simulink model "TwoSegmentArm_muscles_v002"  (R2024b)
settings: Solver=VariableStepAuto  StartTime=0.0  StopTime=20  RelTol=1e-3  AbsTol=1e-3  EnableMultiTasking=on
model workspace (MAT data in the model file):
  bp_out = [-2.4 1.9]
values from neighbouring files (symbols this model uses):
  Param_Mus_MEE = Library_mtu_simulink_mtu_standard_parameters(Param_Mus_MEE)    [init_muscle_MEE.m]
  Param_Mus_MEF = Library_mtu_simulink_mtu_standard_parameters(Param_Mus_MEF)    [init_muscle_MEF.m]
  Param_Mus_MSA = Library_mtu_simulink_mtu_standard_parameters(Param_Mus_MSA)    [init_muscle_MSA.m]
  Param_Mus_MSR = Library_mtu_simulink_mtu_standard_parameters(Param_Mus_MSR)    [init_muscle_MSR.m]
  random_offset = 0    [ddpg_agent.m]
  Ts = 0.075    [ddpg_agent.m]
undefined symbols (not defined in the file or in its folder): gaussian, X, Y, Z
libraries: sm_lib x22, nesl_utility x15, Library_mtu_simulink x8, simulink x8, rllib x1
settings Model: Creator=Isabell  LastModifiedBy=morit
settings SolverCC: AutoScaleAbsTol=off  AlgebraicLoopSolver=TrustRegion
settings DataIOCC: LimitDataPoints=on  MaxDataPoints=10000
settings OptimizationCC: LifeSpan=inf
settings DebuggingCC: UnconnectedInputMsg=warning  UnconnectedOutputMsg=warning  UnconnectedLineMsg=warning  AllowSymbolicDim=off  SFUnexpectedBacktrackingDiag=warning  SFNoUnconditionalDefaultTransitionDiag=warning  SFExecutionAtInitializationDiag=none  ArithmeticOperatorsInVariantConditions=warning
settings ModelReferenceCC: EnableRefExpFcnMdlSchedulingChecks=on
settings SFSimCC: SimUseLocalCustomCode=off  CustomCodeUndefinedFunction=UseInterfaceOnly
settings RTWCC: RTWUseLocalCustomCode=off  GPUComputeCapability=3.5  DLArmComputeVersion=19.05
settings CodeAppCC: StateflowObjectComments=on
settings GRTTargetCC: TargetLangStandard=C89/C90 (ANSI)
settings ConfigComp: CovMetricSettings=dw  CovSaveCumulativeToWorkspaceVar=on  CovSaveSingleToWorkspaceVar=on  CovExternalEMLEnable=off  CovSFcnEnable=off
settings SimscapeCC: SimscapeLogType=all  SimscapeLogSimulationStatistics=on  SimscapeLogDataHistory=10000

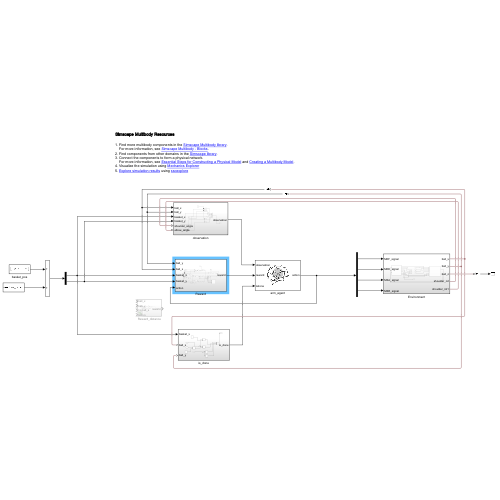
[thumbnail: Simulink's stored preview of the top-level diagram]
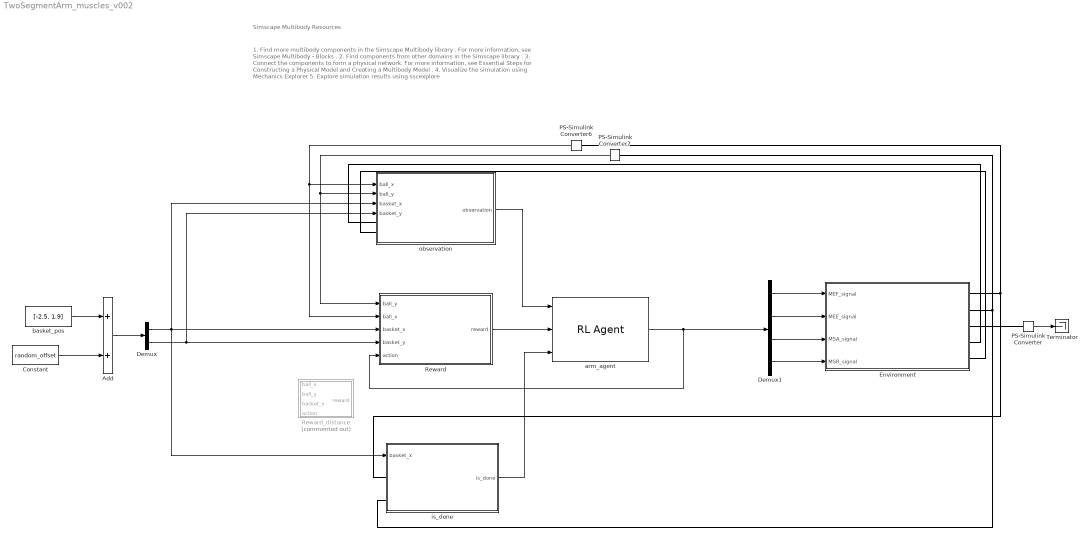
== system TwoSegmentArm_muscles_v002 ==
  note: 1. Find more multibody components in the Simscape Multibody library .
      | For more information, see Simscape Multibody - Blocks .
      | 2. Find components from other domains in the Simscape library .
      | 3. Connect the components to form a physical network.
      | For more information, see Essential Steps for Constructing a Physical Model and Creating a Multibody Model .
      | 4. Visualize the simulation using Mechanics Explorer
      | 5. Explore simulation results using sscexplore
  note: Simscape Multibody Resources
  Add : Sum
  Constant : Constant  Value=random_offset
  Demux : Demux  Outputs=2
  Demux1 : Demux
  Environment : Subsystem
  PS-Simulink Converter : nesl_utility/PS-Simulink Converter  PhysicalDomain=network_engine_domain  SubClassName=ps_output  LeftPortType=input  RightPortType=output  PseudoPeriodic=off  Frequencies=[]  VectorFormat=inherit  Unit=inherit  AffineConversion=off
  PS-Simulink Converter6 : nesl_utility/PS-Simulink Converter  PhysicalDomain=network_engine_domain  SubClassName=ps_output  LeftPortType=input  RightPortType=output  PseudoPeriodic=off  Frequencies=[]  VectorFormat=inherit  Unit=inherit  AffineConversion=off
  PS-Simulink Converter7 : nesl_utility/PS-Simulink Converter  PhysicalDomain=network_engine_domain  SubClassName=ps_output  LeftPortType=input  RightPortType=output  PseudoPeriodic=off  Frequencies=[]  VectorFormat=inherit  Unit=inherit  AffineConversion=off
  Reward : Subsystem
  Reward_distance : Subsystem  Commented=on
  Terminator : Terminator
  arm_agent : rllib/RL Agent  Agent=agent  ExternalActionAsInput=off  ProvideLastAction=off  ProvideCumRwd=off  TreatAsDirectFeedthrough=on  UseStrictObservationDataTypes=off
  basket_pos : Constant  Value=[-2.5, 1.9]
  is_done : Subsystem
  observation : Subsystem
  wires:
  basket_pos/1 -> Add/1
  Add/1 -> Demux/1
  Demux1/3 -> Environment/3(MSA_signal)
  Demux1/2 -> Environment/2(MEE_signal)
  Constant/1 -> Add/2
  Demux1/1 -> Environment/1(MEF_signal)
  Demux1/4 -> Environment/4(MSR_signal)
  PS-Simulink Converter/1 -> Terminator/1
  observation/1(observation) -> arm_agent/1
  Demux/2 -> observation/4(basket_y), Reward/4(basket_y)
  Demux/1 -> Reward/3(basket_x), observation/3(basket_x), is_done/1(basket_x)
  is_done/1(is_done) -> arm_agent/3
  Reward/1(reward) -> arm_agent/2
  PS-Simulink Converter7/1 -> observation/2(ball_y), Reward/1(ball_y)
  arm_agent/1 -> Reward/5(action), Demux1/1
  PS-Simulink Converter6/1 -> Reward/2(ball_x), observation/1(ball_x)
  connections:
  Environment/RConn3 -- PS-Simulink Converter/LConn1
  Environment/RConn5 -- observation/LConn2
  Environment/RConn4 -- observation/LConn1
  Environment/RConn1 -- PS-Simulink Converter6/LConn1 -- is_done/LConn1
  PS-Simulink Converter7/LConn1 -- is_done/LConn2 -- Environment/RConn2

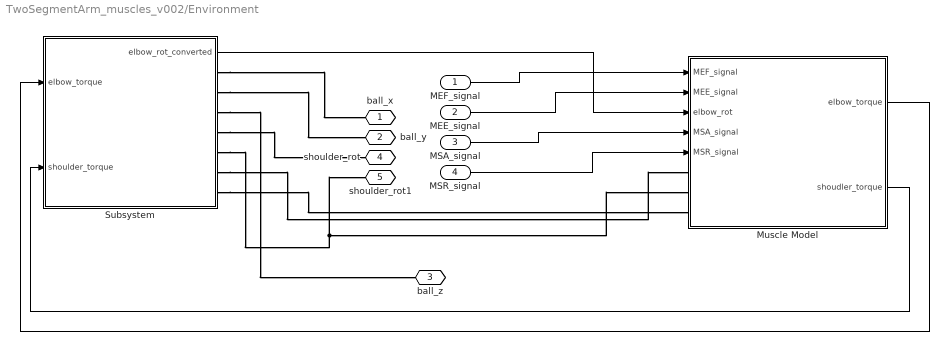
== system TwoSegmentArm_muscles_v002/Environment ==
  MEF_signal : Inport
  MEE_signal : Inport  Port=2
  MSA_signal : Inport  Port=3
  MSR_signal : Inport  Port=4
  Muscle Model : Subsystem
  Subsystem : Subsystem
  ball_x : PMIOPort  Side=Right
  ball_y : PMIOPort  Port=2  Side=Right
  ball_z : PMIOPort  Port=3  Side=Right
  shoulder_rot : PMIOPort  Port=4  Side=Right
  shoulder_rot1 : PMIOPort  Port=5  Side=Right
  wires:
  Muscle Model/2(shoudler_torque) -> Subsystem/2(shoulder_torque)
  Subsystem/1(elbow_rot_converted) -> Muscle Model/3(elbow_rot)
  MEF_signal/1 -> Muscle Model/1(MEF_signal)
  Muscle Model/1(elbow_torque) -> Subsystem/1(elbow_torque)
  MSA_signal/1 -> Muscle Model/4(MSA_signal)
  MSR_signal/1 -> Muscle Model/5(MSR_signal)
  MEE_signal/1 -> Muscle Model/2(MEE_signal)
  connections:
  Subsystem/RConn7 -- Muscle Model/LConn3
  Subsystem/RConn5 -- shoulder_rot1/RConn1 -- Muscle Model/LConn2
  Subsystem/RConn3 -- ball_z/RConn1
  Subsystem/RConn2 -- ball_y/RConn1
  Subsystem/RConn6 -- Muscle Model/LConn1
  Subsystem/RConn1 -- ball_x/RConn1
  Subsystem/RConn4 -- shoulder_rot/RConn1

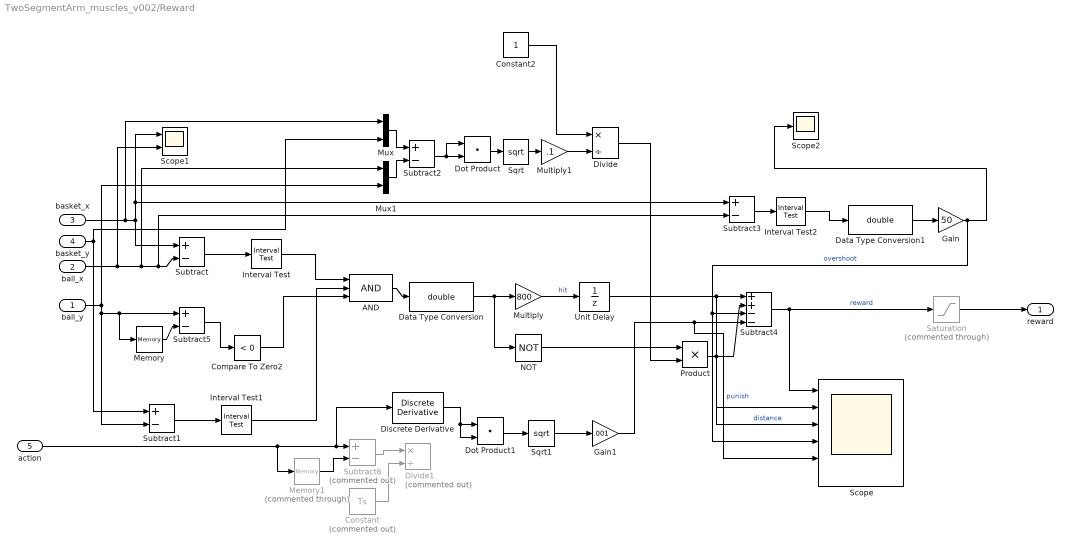
== system TwoSegmentArm_muscles_v002/Reward ==
  ball_y : Inport
  ball_x : Inport  Port=2
  basket_x : Inport  Port=3
  basket_y : Inport  Port=4
  action : Inport  Port=5
  AND : Logic  Inputs=3  IconShape=distinctive  AllPortsSameDT=off  OutDataTypeStr=boolean
  Compare To Zero2 : simulink/Logic and Bit Operations/Compare To Zero  relop=<  OutDataTypeStr=boolean
  Constant : Constant  Commented=on  Value=Ts
  Constant2 : Constant
  Data Type Conversion : DataTypeConversion  OutDataTypeStr=double  SaturateOnIntegerOverflow=off  RndMeth=Floor
  Data Type Conversion1 : DataTypeConversion  OutDataTypeStr=double  SaturateOnIntegerOverflow=off  RndMeth=Floor
  Discrete Derivative : simulink/Discrete/Discrete Derivative  gainval=1.0  ICPrevScaledInput=0.0  OutMin=[]  OutMax=[]  OutDataType=fixdt(1, 16)  OutScaling=2^-10  DoSatur=off
  Divide : Product  Inputs=*/
  Divide1 : Product  Commented=on  Inputs=*/
  Dot Product : DotProduct  OutDataTypeStr=Inherit: Inherit via internal rule
  Dot Product1 : DotProduct  OutDataTypeStr=Inherit: Inherit via internal rule
  Gain : Gain  Gain=50
  Gain1 : Gain  Gain=.001
  Interval Test : simulink/Logic and Bit Operations/Interval Test  IntervalClosedRight=on  uplimit=0.25  IntervalClosedLeft=on  lowlimit=-0.25  OutDataTypeStr=boolean
  Interval Test1 : simulink/Logic and Bit Operations/Interval Test  IntervalClosedRight=on  uplimit=0.05  IntervalClosedLeft=on  lowlimit=-0.25  OutDataTypeStr=boolean
  Interval Test2 : simulink/Logic and Bit Operations/Interval Test  IntervalClosedRight=on  uplimit=0.85  IntervalClosedLeft=on  lowlimit=0.25  OutDataTypeStr=boolean
  Memory : Memory
  Memory1 : Memory  Commented=through
  Multiply : Gain  Gain=800
  Multiply1 : Gain  Gain=.1
  Mux : Mux  Inputs=2
  Mux1 : Mux  Inputs=2
  NOT : Logic  Operator=NOT  IconShape=distinctive  AllPortsSameDT=off  OutDataTypeStr=boolean
  Product : Product
  Saturation : Saturate  Commented=through  UpperLimit=1500  LowerLimit=-500
  Scope : Scope  NumInputPorts=6
  Scope1 : Scope  NumInputPorts=2
  Scope2 : Scope
  Sqrt : Sqrt
  Sqrt1 : Sqrt
  Subtract{,1..3,5} (5 alike) : Sum  Inputs=+-
  Subtract4 : Sum  Inputs=++--
  Subtract6 : Sum  Commented=on  Inputs=+-
  Unit Delay : UnitDelay  SampleTime=-1  HasFrameUpgradeWarning=on
  reward : Outport
  wires:
  basket_x/1 -> Mux/1, Subtract/1, Subtract3/1, Scope1/1
  ball_x/1 -> Scope1/2, Mux1/1, Subtract3/2, Subtract/2
  Subtract/1 -> Interval Test/1
  ball_y/1 -> Subtract1/2, Memory/1, Subtract5/1, Mux1/2
  Subtract5/1 -> Compare To Zero2/1
  basket_y/1 -> Subtract1/1, Mux/2
  AND/1 -> Data Type Conversion/1
  NOT/1 -> Product/1
  Multiply/1 -> Unit Delay/1  "hit"
  Product/1 -> Subtract4/2, Scope/3  "distance"
  Subtract4/1 -> Saturation/1, Scope/1  "reward"
  Data Type Conversion/1 -> NOT/1, Multiply/1
  Interval Test/1 -> AND/1
  Subtract1/1 -> Interval Test1/1
  Interval Test1/1 -> AND/2
  Mux/1 -> Subtract2/1
  Mux1/1 -> Subtract2/2
  Subtract2/1 -> Dot Product/2, Dot Product/1
  Dot Product/1 -> Sqrt/1
  Sqrt/1 -> Multiply1/1
  Subtract3/1 -> Interval Test2/1
  Interval Test2/1 -> Data Type Conversion1/1
  Data Type Conversion1/1 -> Gain/1
  Gain/1 -> Scope/4, Subtract4/3, Scope2/1  "overshoot"
  Dot Product1/1 -> Sqrt1/1
  Gain1/1 -> Scope/5, Subtract4/4  "punish"
  Constant2/1 -> Divide/1
  Multiply1/1 -> Divide/2
  Divide/1 -> Product/2
  Sqrt1/1 -> Gain1/1
  Unit Delay/1 -> Scope/2, Subtract4/1
  Compare To Zero2/1 -> AND/3
  Memory/1 -> Subtract5/2
  Saturation/1 -> reward/1
  action/1 -> Memory1/1, Discrete Derivative/1, Subtract6/1
  Subtract6/1 -> Divide1/1
  Memory1/1 -> Subtract6/2
  Constant/1 -> Divide1/2
  Discrete Derivative/1 -> Dot Product1/2, Dot Product1/1

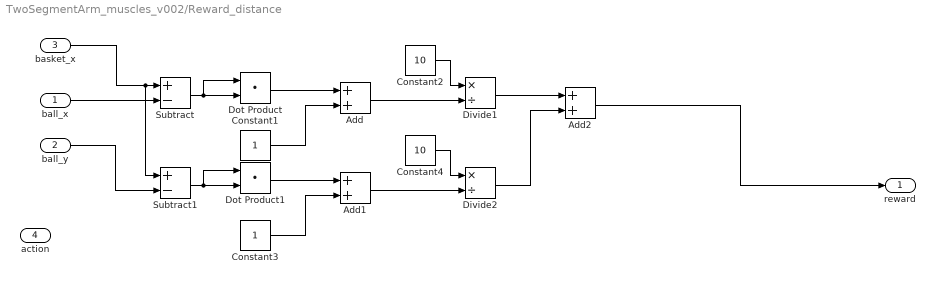
== system TwoSegmentArm_muscles_v002/Reward_distance ==
  ball_x : Inport
  ball_y : Inport  Port=2
  basket_x : Inport  Port=3
  action : Inport  Port=4
  Add : Sum
  Add1 : Sum
  Add2 : Sum
  Constant1 : Constant
  Constant2 : Constant  Value=10
  Constant3 : Constant
  Constant4 : Constant  Value=10
  Divide1 : Product  Inputs=*/
  Divide2 : Product  Inputs=*/
  Dot Product : DotProduct  OutDataTypeStr=Inherit: Inherit via internal rule
  Dot Product1 : DotProduct  OutDataTypeStr=Inherit: Inherit via internal rule
  Subtract : Sum  Inputs=+-
  Subtract1 : Sum  Inputs=+-
  reward : Outport
  wires:
  Add/1 -> Divide1/2
  Constant2/1 -> Divide1/1
  Subtract/1 -> Dot Product/1, Dot Product/2
  ball_x/1 -> Subtract/2
  Dot Product/1 -> Add/1
  Constant1/1 -> Add/2
  basket_x/1 -> Subtract1/1, Subtract/1
  Divide1/1 -> Add2/1
  Add1/1 -> Divide2/2
  Constant4/1 -> Divide2/1
  Dot Product1/1 -> Add1/1
  Subtract1/1 -> Dot Product1/1, Dot Product1/2
  Constant3/1 -> Add1/2
  Add2/1 -> reward/1
  Divide2/1 -> Add2/2
  ball_y/1 -> Subtract1/2

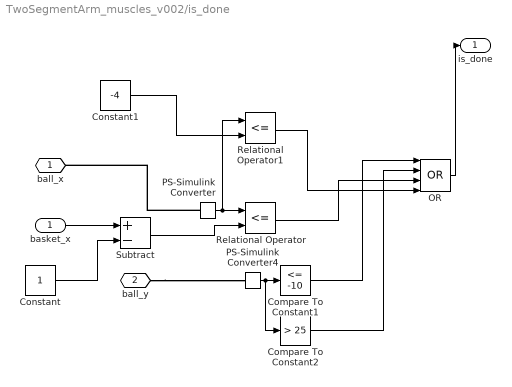
== system TwoSegmentArm_muscles_v002/is_done ==
  basket_x : Inport
  Compare To Constant1 : simulink/Logic and Bit Operations/Compare To Constant  relop=<=  const=-10  OutDataTypeStr=boolean
  Compare To Constant2 : simulink/Logic and Bit Operations/Compare To Constant  relop=>  const=25  OutDataTypeStr=boolean
  Constant : Constant
  Constant1 : Constant  Value=-4
  OR : Logic  Operator=OR  Inputs=4  IconShape=distinctive  AllPortsSameDT=off  OutDataTypeStr=boolean
  PS-Simulink Converter : nesl_utility/PS-Simulink Converter  PhysicalDomain=network_engine_domain  SubClassName=ps_output  LeftPortType=input  RightPortType=output  PseudoPeriodic=off  Frequencies=[]  VectorFormat=inherit  Unit=inherit  AffineConversion=off
  PS-Simulink Converter4 : nesl_utility/PS-Simulink Converter  PhysicalDomain=network_engine_domain  SubClassName=ps_output  LeftPortType=input  RightPortType=output  PseudoPeriodic=off  Frequencies=[]  VectorFormat=inherit  Unit=inherit  AffineConversion=off
  Relational Operator : RelationalOperator  Operator=<=  OutDataTypeStr=boolean  RndMeth=Simplest  InputSameDT=off
  Relational Operator1 : RelationalOperator  Operator=<=  OutDataTypeStr=boolean  RndMeth=Simplest  InputSameDT=off
  Subtract : Sum  Inputs=+-
  ball_x : PMIOPort  Side=Left
  ball_y : PMIOPort  Port=2  Side=Left
  is_done : Outport
  wires:
  PS-Simulink Converter4/1 -> Compare To Constant2/1, Compare To Constant1/1
  Compare To Constant1/1 -> OR/1
  Compare To Constant2/1 -> OR/2
  OR/1 -> is_done/1
  PS-Simulink Converter/1 -> Relational Operator1/1, Relational Operator/1
  Relational Operator/1 -> OR/3
  Constant/1 -> Subtract/2
  Subtract/1 -> Relational Operator/2
  basket_x/1 -> Subtract/1
  Constant1/1 -> Relational Operator1/2
  Relational Operator1/1 -> OR/4
  connections:
  ball_y/RConn1 -- PS-Simulink Converter4/LConn1
  PS-Simulink Converter/LConn1 -- ball_x/RConn1

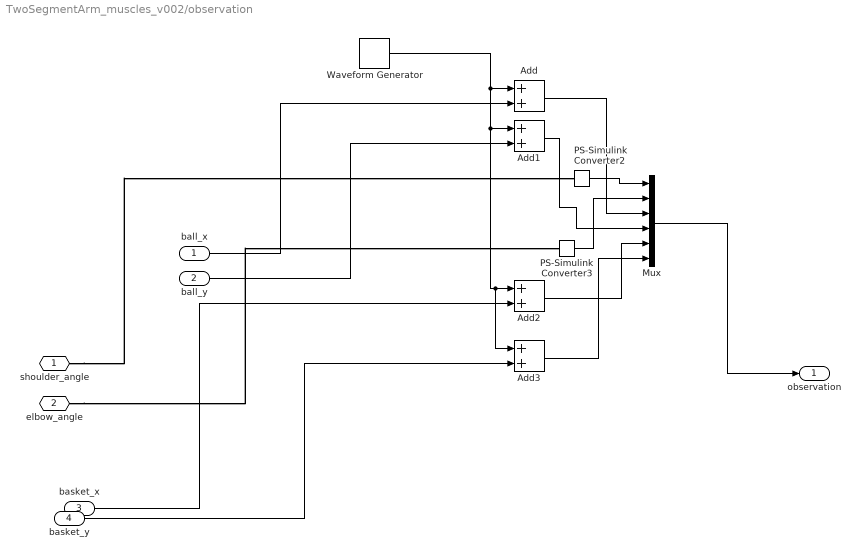
== system TwoSegmentArm_muscles_v002/observation ==
  ball_x : Inport
  ball_y : Inport  Port=2
  basket_x : Inport  Port=3
  basket_y : Inport  Port=4
  Add{,1..3} (4 alike) : Sum
  Mux : Mux  Inputs=6
  PS-Simulink Converter2 : nesl_utility/PS-Simulink Converter  PhysicalDomain=network_engine_domain  SubClassName=ps_output  LeftPortType=input  RightPortType=output  PseudoPeriodic=off  Frequencies=[]  VectorFormat=inherit  Unit=inherit  AffineConversion=off
  PS-Simulink Converter3 : nesl_utility/PS-Simulink Converter  PhysicalDomain=network_engine_domain  SubClassName=ps_output  LeftPortType=input  RightPortType=output  PseudoPeriodic=off  Frequencies=[]  VectorFormat=inherit  Unit=inherit  AffineConversion=off
  Waveform Generator : simulink/Sources/Waveform Generator  OutMin=[]  OutMax=[]  OutDataTypeStr=double  SelectedSignal=1  Signals=gaussian(0, 0, 120)  BlockNames=MultiportSwitch_2798d07791aa46f  SampleTime=0.1
  shoulder_angle : PMIOPort  Side=Left
  elbow_angle : PMIOPort  Port=2  Side=Left
  observation : Outport
  wires:
  Add/1 -> Mux/3
  Add1/1 -> Mux/4
  Waveform Generator/1 -> Add3/1, Add2/1, Add1/1, Add/1
  PS-Simulink Converter3/1 -> Mux/2
  Add3/1 -> Mux/6
  PS-Simulink Converter2/1 -> Mux/1
  Add2/1 -> Mux/5
  basket_y/1 -> Add3/2
  ball_x/1 -> Add/2
  Mux/1 -> observation/1
  ball_y/1 -> Add1/2
  basket_x/1 -> Add2/2
  connections:
  elbow_angle/RConn1 -- PS-Simulink Converter3/LConn1
  shoulder_angle/RConn1 -- PS-Simulink Converter2/LConn1

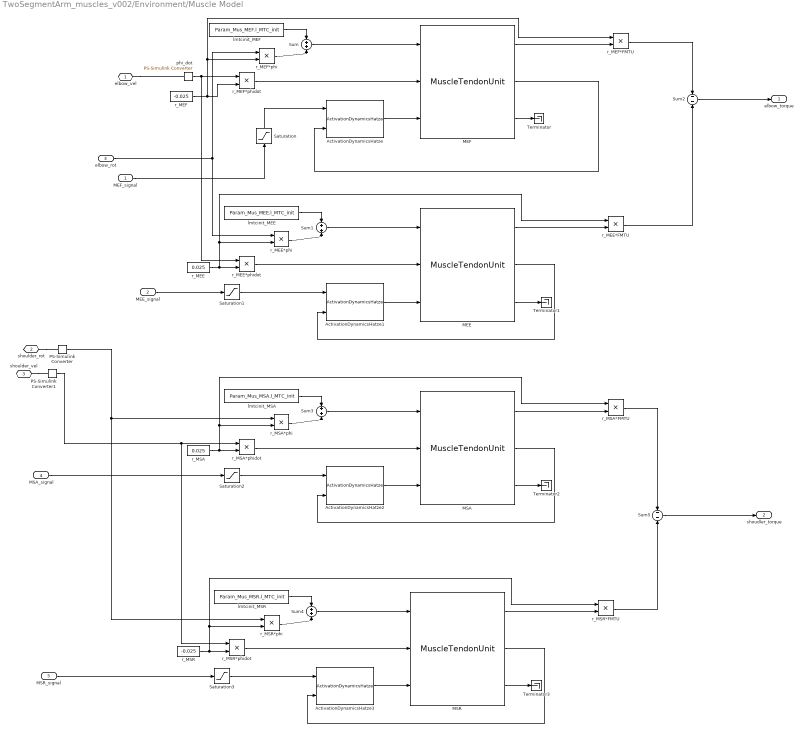
== system TwoSegmentArm_muscles_v002/Environment/Muscle Model ==
  MEF_signal : Inport
  MEE_signal : Inport  Port=2
  elbow_rot : Inport  Port=3
  MSA_signal : Inport  Port=4
  MSR_signal : Inport  Port=5
  ActivationDynamicsHatze : Library_mtu_simulink/ActivationDynamicsHatze  Act_Param=Param_Mus_MEF.ActDyn  Mus_Param=Param_Mus_MEF
  ActivationDynamicsHatze1 : Library_mtu_simulink/ActivationDynamicsHatze  Act_Param=Param_Mus_MEE.ActDyn  Mus_Param=Param_Mus_MEE
  ActivationDynamicsHatze2 : Library_mtu_simulink/ActivationDynamicsHatze  Act_Param=Param_Mus_MEE.ActDyn  Mus_Param=Param_Mus_MEE
  ActivationDynamicsHatze3 : Library_mtu_simulink/ActivationDynamicsHatze  Act_Param=Param_Mus_MEE.ActDyn  Mus_Param=Param_Mus_MEE
  MEE : Library_mtu_simulink/MuscleTendonUnit  Mus_Param=Param_Mus_MEE
  MEF : Library_mtu_simulink/MuscleTendonUnit  Mus_Param=Param_Mus_MEF
  MSA : Library_mtu_simulink/MuscleTendonUnit  Mus_Param=Param_Mus_MSA
  MSR : Library_mtu_simulink/MuscleTendonUnit  Mus_Param=Param_Mus_MSR
  PS-Simulink Converter : nesl_utility/PS-Simulink Converter  PhysicalDomain=network_engine_domain  SubClassName=ps_output  LeftPortType=input  RightPortType=output  PseudoPeriodic=off  Frequencies=[]  VectorFormat=inherit  Unit=inherit  AffineConversion=off
  PS-Simulink Converter1 : nesl_utility/PS-Simulink Converter  PhysicalDomain=network_engine_domain  SubClassName=ps_output  LeftPortType=input  RightPortType=output  PseudoPeriodic=off  Frequencies=[]  VectorFormat=inherit  Unit=inherit  AffineConversion=off
  Saturation{,1..3} (4 alike) : Saturate  UpperLimit=1  LowerLimit=0
  Sum{,1,3..4} (4 alike) : Sum  Inputs=+|+
  Sum2 : Sum  Inputs=-|-
  Sum5 : Sum  Inputs=-|-
  Terminator{,1..3} (4 alike) : Terminator
  lmtcinit_MEE : Constant  Value=Param_Mus_MEE.l_MTC_init
  lmtcinit_MEF : Constant  Value=Param_Mus_MEF.l_MTC_init
  lmtcinit_MSA : Constant  Value=Param_Mus_MSA.l_MTC_init
  lmtcinit_MSR : Constant  Value=Param_Mus_MSR.l_MTC_init
  phi_dot : nesl_utility/PS-Simulink Converter  PhysicalDomain=network_engine_domain  SubClassName=ps_output  LeftPortType=input  RightPortType=output  PseudoPeriodic=off  Frequencies=[]  VectorFormat=1-D array  Unit=inherit  AffineConversion=off
  r_MEE : Constant  Value=0.025
  r_MEE*FMTU : Product
  r_MEE*phi : Product
  r_MEE*phidot : Product
  r_MEF : Constant  Value=-0.025
  r_MEF*FMTU : Product
  r_MEF*phi : Product
  r_MEF*phidot : Product
  r_MSA : Constant  Value=0.025
  r_MSA*FMTU : Product
  r_MSA*phi : Product
  r_MSA*phidot : Product
  r_MSR : Constant  Value=-0.025
  r_MSR*FMTU : Product
  r_MSR*phi : Product
  r_MSR*phidot : Product
  elbow_vel : PMIOPort  Side=Left
  shoulder_rot : PMIOPort  Port=2  Side=Left
  shoulder_vel : PMIOPort  Port=3  Side=Left
  elbow_torque : Outport
  shoudler_torque : Outport  Port=2
  wires:
  Sum1/1 -> MEE/1
  MEE/3 -> Terminator1/1
  r_MEE*phi/1 -> Sum1/2
  elbow_rot/1 -> r_MEF*phi/1, r_MEE*phi/1
  r_MEF*phi/1 -> Sum/2
  r_MEF*phidot/1 -> MEF/2
  r_MEE/1 -> r_MEE*FMTU/1, r_MEE*phi/2, r_MEE*phidot/2
  MEF/3 -> Terminator/1
  r_MEE*FMTU/1 -> Sum2/2
  Saturation/1 -> ActivationDynamicsHatze/1
  MEE/1 -> r_MEE*FMTU/2
  r_MEF/1 -> r_MEF*FMTU/1, r_MEF*phi/2, r_MEF*phidot/2
  ActivationDynamicsHatze/1 -> MEF/3
  ActivationDynamicsHatze1/1 -> MEE/3
  Saturation1/1 -> ActivationDynamicsHatze1/1
  MEF/2 -> ActivationDynamicsHatze/2
  Sum/1 -> MEF/1
  MEF/1 -> r_MEF*FMTU/2
  MEE_signal/1 -> Saturation1/1
  phi_dot/1 -> r_MEE*phidot/1, r_MEF*phidot/1
  lmtcinit_MEF/1 -> Sum/1
  r_MEF*FMTU/1 -> Sum2/1
  r_MEE*phidot/1 -> MEE/2
  lmtcinit_MEE/1 -> Sum1/1
  MEE/2 -> ActivationDynamicsHatze1/2
  Sum2/1 -> elbow_torque/1
  MEF_signal/1 -> Saturation/1
  MSR/2 -> ActivationDynamicsHatze3/2
  MSR/1 -> r_MSR*FMTU/2
  r_MSR*FMTU/1 -> Sum5/2
  PS-Simulink Converter/1 -> r_MSR*phi/1, r_MSA*phi/1
  r_MSR*phi/1 -> Sum4/2
  PS-Simulink Converter1/1 -> r_MSR*phidot/1, r_MSA*phidot/1
  MSR/3 -> Terminator3/1
  ActivationDynamicsHatze3/1 -> MSR/3
  ActivationDynamicsHatze2/1 -> MSA/3
  Saturation3/1 -> ActivationDynamicsHatze3/1
  r_MSA*phidot/1 -> MSA/2
  r_MSR/1 -> r_MSR*FMTU/1, r_MSR*phi/2, r_MSR*phidot/2
  r_MSA*phi/1 -> Sum3/2
  Sum4/1 -> MSR/1
  MSA/2 -> ActivationDynamicsHatze2/2
  Sum3/1 -> MSA/1
  r_MSA*FMTU/1 -> Sum5/1
  Saturation2/1 -> ActivationDynamicsHatze2/1
  r_MSR*phidot/1 -> MSR/2
  MSA/3 -> Terminator2/1
  lmtcinit_MSR/1 -> Sum4/1
  lmtcinit_MSA/1 -> Sum3/1
  r_MSA/1 -> r_MSA*FMTU/1, r_MSA*phi/2, r_MSA*phidot/2
  MSA/1 -> r_MSA*FMTU/2
  MSA_signal/1 -> Saturation2/1
  MSR_signal/1 -> Saturation3/1
  Sum5/1 -> shoudler_torque/1
  connections:
  elbow_vel/RConn1 -- phi_dot/LConn1
  shoulder_rot/RConn1 -- PS-Simulink Converter/LConn1
  shoulder_vel/RConn1 -- PS-Simulink Converter1/LConn1

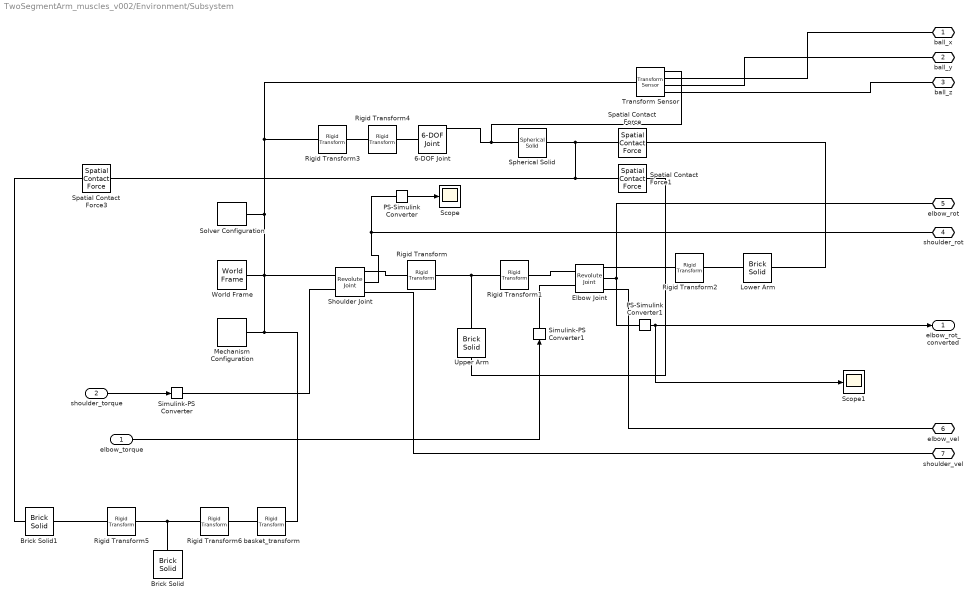
== system TwoSegmentArm_muscles_v002/Environment/Subsystem ==
  elbow_torque : Inport
  shoulder_torque : Inport  Port=2
  6-DOF Joint : sm_lib/Joints/6-DOF Joint  JointMode=Normal  CompositeWrenchDir=FollowerOnBase  CompositeWrenchFrame=BaseFrame  SenseConstraintForce=off  SenseConstraintTorque=off  SenseTotalForce=off  SenseTotalTorque=off  PxPositionTargetSpecify=off  PxPositionTargetPriority=High  PxPositionTargetValue=0  PxPositionTargetValueUnits=m  PxVelocityTargetSpecify=off  PxVelocityTargetPriority=High  PxVelocityTargetValue=0  PxVelocityTargetValueUnits=m/s  PxEquilibriumPosition=0  PxEquilibriumPositionUnits=m  PxSpringStiffness=0  PxSpringStiffnessUnits=N/m  PxDampingCoefficient=0  PxDampingCoefficientUnits=N/(m/s)  PxLowerLimitSpecify=off  PxLowerLimitBound=-1  PxLowerLimitBoundUnits=m  PxLowerLimitStiffness=1e6  PxLowerLimitStiffnessUnits=N/m  PxLowerLimitDamping=1e3  PxLowerLimitDampingUnits=N/(m/s)  PxLowerLimitTransitionRegionWidth=1e-4  PxLowerLimitTransitionRegionWidthUnits=m  PxUpperLimitSpecify=off  PxUpperLimitBound=1  PxUpperLimitBoundUnits=m  PxUpperLimitStiffness=1e6  PxUpperLimitStiffnessUnits=N/m  PxUpperLimitDamping=1e3  PxUpperLimitDampingUnits=N/(m/s)  PxUpperLimitTransitionRegionWidth=1e-4  PxUpperLimitTransitionRegionWidthUnits=m  PxTorqueActuationMode=NoTorque  PxMotionActuationMode=ComputedMotion  PxSensePosition=on  PxSenseVelocity=off  PxSenseAcceleration=off  PxSenseTorqueForce=off  PxSenseLowerLimitTorqueForce=off  PxSenseUpperLimitTorqueForce=off  PyPositionTargetSpecify=off  PyPositionTargetPriority=High  PyPositionTargetValue=0  PyPositionTargetValueUnits=m  PyVelocityTargetSpecify=off  PyVelocityTargetPriority=High  PyVelocityTargetValue=0  PyVelocityTargetValueUnits=m/s  PyEquilibriumPosition=0  PyEquilibriumPositionUnits=m  PySpringStiffness=0  PySpringStiffnessUnits=N/m  PyDampingCoefficient=0  PyDampingCoefficientUnits=N/(m/s)  PyLowerLimitSpecify=off  PyLowerLimitBound=-1  PyLowerLimitBoundUnits=m  PyLowerLimitStiffness=1e6  PyLowerLimitStiffnessUnits=N/m  PyLowerLimitDamping=1e3  PyLowerLimitDampingUnits=N/(m/s)  PyLowerLimitTransitionRegionWidth=1e-4  PyLowerLimitTransitionRegionWidthUnits=m  PyUpperLimitSpecify=off  PyUpperLimitBound=1  PyUpperLimitBoundUnits=m  PyUpperLimitStiffness=1e6  PyUpperLimitStiffnessUnits=N/m  PyUpperLimitDamping=1e3  PyUpperLimitDampingUnits=N/(m/s)  PyUpperLimitTransitionRegionWidth=1e-4  PyUpperLimitTransitionRegionWidthUnits=m  PyTorqueActuationMode=NoTorque  PyMotionActuationMode=ComputedMotion  PySensePosition=on  PySenseVelocity=off  PySenseAcceleration=off  PySenseTorqueForce=off  PySenseLowerLimitTorqueForce=off  PySenseUpperLimitTorqueForce=off  PzPositionTargetSpecify=off  PzPositionTargetPriority=High  PzPositionTargetValue=0  PzPositionTargetValueUnits=m  PzVelocityTargetSpecify=off  PzVelocityTargetPriority=High  PzVelocityTargetValue=0  PzVelocityTargetValueUnits=m/s  PzEquilibriumPosition=0  PzEquilibriumPositionUnits=m  PzSpringStiffness=0  PzSpringStiffnessUnits=N/m  PzDampingCoefficient=0  PzDampingCoefficientUnits=N/(m/s)  PzLowerLimitSpecify=off  PzLowerLimitBound=-1  PzLowerLimitBoundUnits=m  PzLowerLimitStiffness=1e6  PzLowerLimitStiffnessUnits=N/m  PzLowerLimitDamping=1e3  PzLowerLimitDampingUnits=N/(m/s)  PzLowerLimitTransitionRegionWidth=1e-4  PzLowerLimitTransitionRegionWidthUnits=m  PzUpperLimitSpecify=off  PzUpperLimitBound=1  PzUpperLimitBoundUnits=m  PzUpperLimitStiffness=1e6  PzUpperLimitStiffnessUnits=N/m  PzUpperLimitDamping=1e3  PzUpperLimitDampingUnits=N/(m/s)  PzUpperLimitTransitionRegionWidth=1e-4  PzUpperLimitTransitionRegionWidthUnits=m  PzTorqueActuationMode=NoTorque  PzMotionActuationMode=ComputedMotion  PzSensePosition=on  PzSenseVelocity=off  PzSenseAcceleration=off  PzSenseTorqueForce=off  PzSenseLowerLimitTorqueForce=off  PzSenseUpperLimitTorqueForce=off  SphPositionTargetSpecify=off  SphPositionTargetPriority=High  SphPositionTargetRotationMethod=None  SphPositionTargetFollAlignAxisA=+X  SphPositionTargetBaseAlignAxisA=+Y  SphPositionTargetFollAlignAxisB=+Y  SphPositionTargetBaseAlignAxisB=+Z  SphPositionTargetRotationStandardAxis=+Z  SphPositionTargetRotationAngle=0  SphPositionTargetRotationAngleUnits=deg  SphPositionTargetRotationArbitraryAxis=[0 0 1]  SphPositionTargetRotationSequenceAxes=FollowerAxes  SphPositionTargetRotationSequence=XYX  SphPositionTargetRotationSequenceAngles=[0 0 0]  SphPositionTargetRotationSequenceAnglesUnits=deg  SphPositionTargetRotationMatrix=[1 0 0;0 1 0;0 0 1]  SphPositionTargetQuaternion=[1 0 0 0]  SphVelocityTargetSpecify=off  SphVelocityTargetPriority=High  SphVelocityTargetValue=[0 0 0]  SphVelocityTargetValueUnits=deg/s  SphVelocityTargetInFollowerFrame=on  SphEqPosRotationMethod=None  SphEqPosFollAlignAxisA=+X  SphEqPosBaseAlignAxisA=+Y  SphEqPosFollAlignAxisB=+Y  SphEqPosBaseAlignAxisB=+Z  SphEqPosRotationStandardAxis=+Z  SphEqPosRotationAngle=0  SphEqPosRotationAngleUnits=deg  SphEqPosRotationArbitraryAxis=[0 0 1]  SphEqPosRotationSequenceAxes=FollowerAxes  SphEqPosRotationSequence=XYX  SphEqPosRotationSequenceAngles=[0 0 0]  SphEqPosRotationSequenceAnglesUnits=deg  SphEqPosRotationMatrix=[1 0 0;0 1 0;0 0 1]  SphEqPosQuaternion=[1 0 0 0]  SphSpringStiffness=0  SphSpringStiffnessUnits=N*m/deg  SphDampingCoefficient=0  SphDampingCoefficientUnits=N*m/(deg/s)  SphLowerLimitSpecify=off  SphLowerLimitBound=15  SphLowerLimitBoundUnits=deg  SphLowerLimitStiffness=1e4  SphLowerLimitStiffnessUnits=N*m/deg  SphLowerLimitDamping=10  SphLowerLimitDampingUnits=N*m/(deg/s)  SphLowerLimitTransitionRegionWidth=0.1  SphLowerLimitTransitionRegionWidthUnits=deg  SphUpperLimitSpecify=off  SphUpperLimitBound=45  SphUpperLimitBoundUnits=deg  SphUpperLimitStiffness=1e4  SphUpperLimitStiffnessUnits=N*m/deg  SphUpperLimitDamping=10  SphUpperLimitDampingUnits=N*m/(deg/s)  SphUpperLimitTransitionRegionWidth=0.1  SphUpperLimitTransitionRegionWidthUnits=deg  SphTorqueActuationMode=NoTorque  SphActuateTorqueX=off  SphActuateTorqueY=off  SphActuateTorqueZ=off  SphActuateTorque=off  SphActuationFrame=BaseFrame  SphSensePosition=off  SphSenseVelocityX=off  SphSenseVelocityY=off  SphSenseVelocityZ=off  SphSenseVelocity=off  SphSenseAccelerationX=off  SphSenseAccelerationY=off  SphSenseAccelerationZ=off  SphSenseAcceleration=off  SphSenseLowerLimitTorqueMag=off  SphSenseUpperLimitTorqueMag=off  SphSensingFrame=BaseFrame
  Brick Solid : sm_lib/Body Elements/Brick Solid  BrickDimensions=[.25 .05 .25]  BrickDimensionsUnits=m  ExportEntireGeometry=off  InertiaType=CalculateFromGeometry  BasedOnType=Density  Density=1000  DensityUnits=kg/m^3  Mass=1  MassUnits=kg  CenterOfMass=[0 0 0]  CenterOfMassUnits=m  MomentsOfInertia=[1 1 1]  MomentsOfInertiaUnits=kg*m^2  ProductsOfInertia=[0 0 0]  ProductsOfInertiaUnits=kg*m^2  GraphicType=FromGeometry  MarkerShape=Sphere  MarkerSize=10  GraphicVisPropType=SimpleVisualProperties  GraphicDiffuseColor=[0.5 0.5 0.5]  GraphicOpacity=1  GraphicSpecularColor=[0.5 0.5 0.5 1.0]  GraphicAmbientColor=[0.15 0.15 0.15 1.0]  GraphicEmissiveColor=[0.0 0.0 0.0 1.0]  GraphicShininess=75  DoExposeReferenceFrame=on  SerializedFrames=<Frames/>
  Brick Solid1 : sm_lib/Body Elements/Brick Solid  BrickDimensions=[.05 .3 .3]  BrickDimensionsUnits=m  ExportEntireGeometry=on  InertiaType=CalculateFromGeometry  BasedOnType=Density  Density=1000  DensityUnits=kg/m^3  Mass=1  MassUnits=kg  CenterOfMass=[0 0 0]  CenterOfMassUnits=m  MomentsOfInertia=[1 1 1]  MomentsOfInertiaUnits=kg*m^2  ProductsOfInertia=[0 0 0]  ProductsOfInertiaUnits=kg*m^2  GraphicType=FromGeometry  MarkerShape=Sphere  MarkerSize=10  GraphicVisPropType=SimpleVisualProperties  GraphicDiffuseColor=[0.5 0.5 0.5]  GraphicOpacity=1  GraphicSpecularColor=[0.5 0.5 0.5 1.0]  GraphicAmbientColor=[0.15 0.15 0.15 1.0]  GraphicEmissiveColor=[0.0 0.0 0.0 1.0]  GraphicShininess=75  DoExposeReferenceFrame=on  SerializedFrames=<Frames/>
  Elbow Joint : sm_lib/Joints/Revolute Joint  JointMode=Normal  CompositeWrenchDir=FollowerOnBase  CompositeWrenchFrame=BaseFrame  SenseConstraintForce=off  SenseConstraintTorque=off  SenseTotalForce=off  SenseTotalTorque=off  PositionTargetSpecify=on  PositionTargetPriority=High  PositionTargetValue=-130  PositionTargetValueUnits=deg  VelocityTargetSpecify=off  VelocityTargetPriority=High  VelocityTargetValue=0  VelocityTargetValueUnits=deg/s  EquilibriumPosition=0  EquilibriumPositionUnits=deg  SpringStiffness=0  SpringStiffnessUnits=N*m/deg  DampingCoefficient=0  DampingCoefficientUnits=N*m/(deg/s)  LowerLimitSpecify=on  LowerLimitBound=-135  LowerLimitBoundUnits=deg  LowerLimitStiffness=1000  LowerLimitStiffnessUnits=N*m/deg  LowerLimitDamping=10  LowerLimitDampingUnits=N*m/(rad/s)  LowerLimitTransitionRegionWidth=0.1  LowerLimitTransitionRegionWidthUnits=deg  UpperLimitSpecify=on  UpperLimitBound=0  UpperLimitBoundUnits=deg  UpperLimitStiffness=1000  UpperLimitStiffnessUnits=N*m/rad  UpperLimitDamping=10  UpperLimitDampingUnits=N*m/(rad/s)  UpperLimitTransitionRegionWidth=0.1  UpperLimitTransitionRegionWidthUnits=deg  TorqueActuationMode=InputTorque  MotionActuationMode=ComputedMotion  SensePosition=on  SenseVelocity=on  SenseAcceleration=off  SenseTorqueForce=off  SenseLowerLimitTorqueForce=off  SenseUpperLimitTorqueForce=off
  Lower Arm : sm_lib/Body Elements/Brick Solid  BrickDimensions=[0.01 0.263 0.01]  BrickDimensionsUnits=m  ExportEntireGeometry=on  InertiaType=Custom  BasedOnType=Density  Density=1000  DensityUnits=kg/m^3  Mass=1.65  MassUnits=kg  CenterOfMass=[0 -0.0475 0]  CenterOfMassUnits=m  MomentsOfInertia=[0 0 0.025]  MomentsOfInertiaUnits=kg*m^2  ProductsOfInertia=[0 0 0]  ProductsOfInertiaUnits=kg*m^2  GraphicType=FromGeometry  MarkerShape=Sphere  MarkerSize=10  GraphicVisPropType=SimpleVisualProperties  GraphicDiffuseColor=[0.0 0.0 1.0]  GraphicOpacity=1.0  GraphicSpecularColor=[0.5 0.5 0.5 1.0]  GraphicAmbientColor=[0.15 0.15 0.15 1.0]  GraphicEmissiveColor=[0.0 0.0 0.0 1.0]  GraphicShininess=75  DoExposeReferenceFrame=on  SerializedFrames=<Frames/>
  Mechanism Configuration : sm_lib/Utilities/Mechanism Configuration  UniformGravity=Constant  GravityVector=[0 -9.80665 0]  GravityVectorUnits=m/s^2  LinearizationDelta=0.001  JointModeTransitionNonlinearIterations=2
  PS-Simulink Converter : nesl_utility/PS-Simulink Converter  PhysicalDomain=network_engine_domain  SubClassName=ps_output  LeftPortType=input  RightPortType=output  PseudoPeriodic=off  Frequencies=[]  VectorFormat=1-D array  Unit=inherit  AffineConversion=off
  PS-Simulink Converter1 : nesl_utility/PS-Simulink Converter  PhysicalDomain=network_engine_domain  SubClassName=ps_output  LeftPortType=input  RightPortType=output  PseudoPeriodic=off  Frequencies=[]  VectorFormat=1-D array  Unit=inherit  AffineConversion=off
  Rigid Transform : sm_lib/Frames and Transforms/Rigid Transform  RotationMethod=None  FollAlignAxisA=+X  BaseAlignAxisA=+Y  FollAlignAxisB=+Y  BaseAlignAxisB=+Z  RotationStandardAxis=+Z  RotationAngle=0.0  RotationAngleUnits=deg  RotationArbitraryAxis=[0 0 1]  RotationSequenceAxes=FollowerAxes  RotationSequence=XYX  RotationSequenceAngles=[0 0 0]  RotationSequenceAnglesUnits=deg  RotationMatrix=[1 0 0; 0 1 0; 0 0 1]  Quaternion=[1 0 0 0]  TranslationMethod=StandardAxis  TranslationCartesianOffset=[0 0 0]  TranslationCartesianOffsetUnits=m  TranslationStandardAxis=+Y  TranslationStandardOffset=-0.1675  TranslationStandardOffsetUnits=m  TranslationROffset=0  TranslationROffsetUnits=m  TranslationThetaOffset=0  TranslationThetaOffsetUnits=deg  TranslationZOffset=0  TranslationZOffsetUnits=m
  Rigid Transform1 : sm_lib/Frames and Transforms/Rigid Transform  RotationMethod=None  FollAlignAxisA=+X  BaseAlignAxisA=+Y  FollAlignAxisB=+Y  BaseAlignAxisB=+Z  RotationStandardAxis=+Z  RotationAngle=0.0  RotationAngleUnits=deg  RotationArbitraryAxis=[0 0 1]  RotationSequenceAxes=FollowerAxes  RotationSequence=XYX  RotationSequenceAngles=[0 0 0]  RotationSequenceAnglesUnits=deg  RotationMatrix=[1 0 0; 0 1 0; 0 0 1]  Quaternion=[1 0 0 0]  TranslationMethod=StandardAxis  TranslationCartesianOffset=[0 0 0]  TranslationCartesianOffsetUnits=m  TranslationStandardAxis=+Y  TranslationStandardOffset=-0.1675  TranslationStandardOffsetUnits=m  TranslationROffset=0  TranslationROffsetUnits=m  TranslationThetaOffset=0  TranslationThetaOffsetUnits=deg  TranslationZOffset=0  TranslationZOffsetUnits=m
  Rigid Transform2 : sm_lib/Frames and Transforms/Rigid Transform  RotationMethod=None  FollAlignAxisA=+X  BaseAlignAxisA=+Y  FollAlignAxisB=+Y  BaseAlignAxisB=+Z  RotationStandardAxis=+Z  RotationAngle=0.0  RotationAngleUnits=deg  RotationArbitraryAxis=[0 0 1]  RotationSequenceAxes=FollowerAxes  RotationSequence=XYX  RotationSequenceAngles=[0 0 0]  RotationSequenceAnglesUnits=deg  RotationMatrix=[1 0 0; 0 1 0; 0 0 1]  Quaternion=[1 0 0 0]  TranslationMethod=StandardAxis  TranslationCartesianOffset=[0 0 0]  TranslationCartesianOffsetUnits=m  TranslationStandardAxis=+Y  TranslationStandardOffset=-0.1315  TranslationStandardOffsetUnits=m  TranslationROffset=0  TranslationROffsetUnits=m  TranslationThetaOffset=0  TranslationThetaOffsetUnits=deg  TranslationZOffset=0  TranslationZOffsetUnits=m
  Rigid Transform3 : sm_lib/Frames and Transforms/Rigid Transform  RotationMethod=None  FollAlignAxisA=+X  BaseAlignAxisA=+Y  FollAlignAxisB=+Y  BaseAlignAxisB=+Z  RotationStandardAxis=+Z  RotationAngle=0  RotationAngleUnits=deg  RotationArbitraryAxis=[0 0 1]  RotationSequenceAxes=FollowerAxes  RotationSequence=XYX  RotationSequenceAngles=[0 0 0]  RotationSequenceAnglesUnits=deg  RotationMatrix=[1 0 0;0 1 0;0 0 1]  Quaternion=[1 0 0 0]  TranslationMethod=StandardAxis  TranslationCartesianOffset=[0 0 0]  TranslationCartesianOffsetUnits=m  TranslationStandardAxis=+X  TranslationStandardOffset=0  TranslationStandardOffsetUnits=m  TranslationROffset=0  TranslationROffsetUnits=m  TranslationThetaOffset=0  TranslationThetaOffsetUnits=deg  TranslationZOffset=0  TranslationZOffsetUnits=m
  Rigid Transform4 : sm_lib/Frames and Transforms/Rigid Transform  RotationMethod=None  FollAlignAxisA=+X  BaseAlignAxisA=+Y  FollAlignAxisB=+Y  BaseAlignAxisB=+Z  RotationStandardAxis=+Z  RotationAngle=0  RotationAngleUnits=deg  RotationArbitraryAxis=[0 0 1]  RotationSequenceAxes=FollowerAxes  RotationSequence=XYX  RotationSequenceAngles=[0 0 0]  RotationSequenceAnglesUnits=deg  RotationMatrix=[1 0 0;0 1 0;0 0 1]  Quaternion=[1 0 0 0]  TranslationMethod=StandardAxis  TranslationCartesianOffset=[0 0 0]  TranslationCartesianOffsetUnits=m  TranslationStandardAxis=+Y  TranslationStandardOffset=.33  TranslationStandardOffsetUnits=m  TranslationROffset=0  TranslationROffsetUnits=m  TranslationThetaOffset=0  TranslationThetaOffsetUnits=deg  TranslationZOffset=0  TranslationZOffsetUnits=m
  Rigid Transform5 : sm_lib/Frames and Transforms/Rigid Transform  RotationMethod=None  FollAlignAxisA=+X  BaseAlignAxisA=+Y  FollAlignAxisB=+Y  BaseAlignAxisB=+Z  RotationStandardAxis=+Z  RotationAngle=0  RotationAngleUnits=deg  RotationArbitraryAxis=[0 0 1]  RotationSequenceAxes=FollowerAxes  RotationSequence=XYX  RotationSequenceAngles=[0 0 0]  RotationSequenceAnglesUnits=deg  RotationMatrix=[1 0 0;0 1 0;0 0 1]  Quaternion=[1 0 0 0]  TranslationMethod=Cartesian  TranslationCartesianOffset=[0.19, -0.15,0]  TranslationCartesianOffsetUnits=m  TranslationStandardAxis=-X  TranslationStandardOffset=.3  TranslationStandardOffsetUnits=m  TranslationROffset=0  TranslationROffsetUnits=m  TranslationThetaOffset=0  TranslationThetaOffsetUnits=deg  TranslationZOffset=0  TranslationZOffsetUnits=m
  Rigid Transform6 : sm_lib/Frames and Transforms/Rigid Transform  RotationMethod=None  FollAlignAxisA=+X  BaseAlignAxisA=+Y  FollAlignAxisB=+Y  BaseAlignAxisB=+Z  RotationStandardAxis=+Z  RotationAngle=0  RotationAngleUnits=deg  RotationArbitraryAxis=[0 0 1]  RotationSequenceAxes=FollowerAxes  RotationSequence=XYX  RotationSequenceAngles=[0 0 0]  RotationSequenceAnglesUnits=deg  RotationMatrix=[1 0 0;0 1 0;0 0 1]  Quaternion=[1 0 0 0]  TranslationMethod=StandardAxis  TranslationCartesianOffset=[0 0 0]  TranslationCartesianOffsetUnits=m  TranslationStandardAxis=-X  TranslationStandardOffset=random_offset  TranslationStandardOffsetUnits=m  TranslationROffset=0  TranslationROffsetUnits=m  TranslationThetaOffset=0  TranslationThetaOffsetUnits=deg  TranslationZOffset=0  TranslationZOffsetUnits=m
  Scope : Scope
  Scope1 : Scope
  Shoulder Joint : sm_lib/Joints/Revolute Joint  JointMode=Normal  CompositeWrenchDir=FollowerOnBase  CompositeWrenchFrame=BaseFrame  SenseConstraintForce=off  SenseConstraintTorque=off  SenseTotalForce=off  SenseTotalTorque=off  PositionTargetSpecify=on  PositionTargetPriority=High  PositionTargetValue=-140  PositionTargetValueUnits=deg  VelocityTargetSpecify=off  VelocityTargetPriority=High  VelocityTargetValue=0  VelocityTargetValueUnits=deg/s  EquilibriumPosition=0  EquilibriumPositionUnits=deg  SpringStiffness=0  SpringStiffnessUnits=N*m/deg  DampingCoefficient=0  DampingCoefficientUnits=N*m/(deg/s)  LowerLimitSpecify=on  LowerLimitBound=-180  LowerLimitBoundUnits=deg  LowerLimitStiffness=1000  LowerLimitStiffnessUnits=N*m/rad  LowerLimitDamping=10  LowerLimitDampingUnits=N*m/(rad/s)  LowerLimitTransitionRegionWidth=0.1  LowerLimitTransitionRegionWidthUnits=deg  UpperLimitSpecify=on  UpperLimitBound=0  UpperLimitBoundUnits=deg  UpperLimitStiffness=1000  UpperLimitStiffnessUnits=N*m/rad  UpperLimitDamping=10  UpperLimitDampingUnits=N*m/(rad/s)  UpperLimitTransitionRegionWidth=0.1  UpperLimitTransitionRegionWidthUnits=deg  TorqueActuationMode=InputTorque  MotionActuationMode=ComputedMotion  SensePosition=on  SenseVelocity=on  SenseAcceleration=off  SenseTorqueForce=off  SenseLowerLimitTorqueForce=off  SenseUpperLimitTorqueForce=off
  Simulink-PS Converter : nesl_utility/Simulink-PS Converter  PhysicalDomain=network_engine_domain  SubClassName=ps_input  LeftPortType=input  RightPortType=output  PseudoPeriodic=off  Frequencies=[]  NoiseDistribution=none  NoiseParameters=[]  Unit=1  AffineConversion=off  FilteringAndDerivatives=provide  SimscapeFilterOrder=1  InputFilterTimeConstant=0.001  UdotUserProvided=0
  Simulink-PS Converter1 : nesl_utility/Simulink-PS Converter  PhysicalDomain=network_engine_domain  SubClassName=ps_input  LeftPortType=input  RightPortType=output  PseudoPeriodic=off  Frequencies=[]  NoiseDistribution=none  NoiseParameters=[]  Unit=N*m  AffineConversion=off  FilteringAndDerivatives=provide  SimscapeFilterOrder=1  InputFilterTimeConstant=0.001  UdotUserProvided=0
  Solver Configuration : nesl_utility/Solver Configuration  PhysicalDomain=network_engine_domain  SubClassName=solver  LeftPortType=input  RightPortType=generic  Tones=[]  Harmonics=[]  SimulateNoise=off  Profile=off  UseLocalSampling=off  EnableSwitchedLinearOptims=on  FrequencyDomain=off  UseCCode=off  RelTol=0.001  AbsTol=1e-06  MinStep=1e-09  ToWorkspace=off  RevertToSquareIcSolve=off  NumHomotopyIterations=100  PhasorMode=off  PhasorModeNumHarmonics=1  ConsistencySolver=NEWTON_FTOL  IndexReductionMethod=DerivativeReplacement  DoDC=off  ResidualTolerance=1e-09  ConsistencyTolSource=GLOBAL  ConsistencyAbsTol=0.001  ConsistencyRelTol=0.001  ConsistencyTolFactor=0.001  UseLocalSolver=off  LocalSolverChoice=NE_BACKWARD_EULER_ADVANCER  ResolveIndetEquations=on  FunctionEvalNumThread=1  LocalSolverSampleTime=0.001  DoFixedCost=off  MaxNonlinIter=3  MaxModeIter=2  ComputeImpulses=off  ImpulseIterations=2  LinearAlgebra=Sparse  LinearAlgebraNumThread=0  EquationFormulation=NE_TIME_EF  DelaysMemoryBudget=1024  AutomaticFiltering=on  FilteringTimeConstant=0.001  PartitionStorageMethod=AS_NEEDED  PartitionMemoryBudget=1024  PartitionMethod=FAST  MultibodyUseLocalSolver=off  MultibodyLocalSolverChoice=ODE1  MultibodyLocalSolverSampleTime=0.001
  Spatial Contact Force : sm_lib/Forces and Torques/Spatial Contact Force  NormalForceType=SmoothSpringDamper  NormalStiffness=1e6  NormalStiffnessUnits=N/m  NormalDamping=1e3  NormalDampingUnits=N/(m/s)  NormalTransitionRegionWidth=1e-4  NormalTransitionRegionWidthUnits=m  FrictionType=SmoothStickSlip  CoefficientOfStaticFriction=0.5  CoefficientOfDynamicFriction=0.3  FrictionalCriticalVelocity=1e-3  FrictionalCriticalVelocityUnits=m/s  SenseContactSignal=off  SensePenetrationDepth=off  SenseSeparationDistance=off  SenseNormalForceMagnitude=off  SenseFrictionalForceMagnitude=off  SenseNormalVelocity=off  SenseTangentialVelocity=off  SenseContactBaseRotation=off  SenseContactBaseTranslation=off  SenseContactFollowerRotation=off  SenseContactFollowerTranslation=off  ZeroCrossDetectContactStartAndEnd=off
  Spatial Contact Force1 : sm_lib/Forces and Torques/Spatial Contact Force  NormalForceType=SmoothSpringDamper  NormalStiffness=1e6  NormalStiffnessUnits=N/m  NormalDamping=1e3  NormalDampingUnits=N/(m/s)  NormalTransitionRegionWidth=1e-4  NormalTransitionRegionWidthUnits=m  FrictionType=SmoothStickSlip  CoefficientOfStaticFriction=0.5  CoefficientOfDynamicFriction=0.3  FrictionalCriticalVelocity=1e-3  FrictionalCriticalVelocityUnits=m/s  SenseContactSignal=off  SensePenetrationDepth=off  SenseSeparationDistance=off  SenseNormalForceMagnitude=off  SenseFrictionalForceMagnitude=off  SenseNormalVelocity=off  SenseTangentialVelocity=off  SenseContactBaseRotation=off  SenseContactBaseTranslation=off  SenseContactFollowerRotation=off  SenseContactFollowerTranslation=off  ZeroCrossDetectContactStartAndEnd=off
  Spatial Contact Force3 : sm_lib/Forces and Torques/Spatial Contact Force  NormalForceType=SmoothSpringDamper  NormalStiffness=1e6  NormalStiffnessUnits=N/m  NormalDamping=1e3  NormalDampingUnits=N/(m/s)  NormalTransitionRegionWidth=1e-4  NormalTransitionRegionWidthUnits=m  FrictionType=SmoothStickSlip  CoefficientOfStaticFriction=0.5  CoefficientOfDynamicFriction=0.3  FrictionalCriticalVelocity=1e-3  FrictionalCriticalVelocityUnits=m/s  SenseContactSignal=off  SensePenetrationDepth=off  SenseSeparationDistance=off  SenseNormalForceMagnitude=off  SenseFrictionalForceMagnitude=off  SenseNormalVelocity=off  SenseTangentialVelocity=off  SenseContactBaseRotation=off  SenseContactBaseTranslation=off  SenseContactFollowerRotation=off  SenseContactFollowerTranslation=off  ZeroCrossDetectContactStartAndEnd=off
  Spherical Solid : sm_lib/Body Elements/Spherical Solid  SphereRadius=0.05  SphereRadiusUnits=m  ExportEntireGeometry=on  InertiaType=Custom  BasedOnType=Density  Density=1000  DensityUnits=kg/m^3  Mass=0.05  MassUnits=kg  CenterOfMass=[0 0 0]  CenterOfMassUnits=m  MomentsOfInertia=[1 1 1]  MomentsOfInertiaUnits=kg*m^2  ProductsOfInertia=[0 0 0]  ProductsOfInertiaUnits=kg*m^2  GraphicType=FromGeometry  MarkerShape=Sphere  MarkerSize=10  GraphicVisPropType=SimpleVisualProperties  GraphicDiffuseColor=[0.5 0.5 0.5]  GraphicOpacity=1  GraphicSpecularColor=[0.5 0.5 0.5 1.0]  GraphicAmbientColor=[0.15 0.15 0.15 1.0]  GraphicEmissiveColor=[0.0 0.0 0.0 1.0]  GraphicShininess=75  DoExposeReferenceFrame=on  SerializedFrames=<Frames/>
  Transform Sensor : sm_lib/Frames and Transforms/Transform Sensor  MeasurementFrame=World  RotationSequence=XYX  SenseAngle=off  SenseAxis=off  SenseQ=off  SenseR=off  SenseRotationSequence=off  SenseOmegaX=off  SenseOmegaY=off  SenseOmegaZ=off  SenseOmega=off  SenseQDot=off  SenseRDot=off  SenseRotationSequenceDot=off  SenseAlphaX=off  SenseAlphaY=off  SenseAlphaZ=off  SenseAlpha=off  SenseQDDot=off  SenseRDDot=off  SenseX=on  SenseY=on  SenseZ=on  SenseXYZ=off  SenseRad=off  SenseAzim=off  SenseDist=off  SenseInc=off  SenseXDot=off  SenseYDot=off  SenseZDot=off  SenseXYZDot=off  SenseRadDot=off  SenseAzimDot=off  SenseDistDot=off  SenseIncDot=off  SenseXDDot=off  SenseYDDot=off  SenseZDDot=off  SenseXYZDDot=off  SenseRadDDot=off  SenseAzimDDot=off  SenseDistDDot=off  SenseIncDDot=off
  Upper Arm : sm_lib/Body Elements/Brick Solid  BrickDimensions=[0.01 0.335 0.01]  BrickDimensionsUnits=m  ExportEntireGeometry=on  InertiaType=Custom  BasedOnType=Density  Density=1000  DensityUnits=kg/m^3  Mass=2.1  MassUnits=kg  CenterOfMass=[0 0.0215 0]  CenterOfMassUnits=m  MomentsOfInertia=[0 0 0.024]  MomentsOfInertiaUnits=kg*m^2  ProductsOfInertia=[0 0 0]  ProductsOfInertiaUnits=kg*m^2  GraphicType=FromGeometry  MarkerShape=Sphere  MarkerSize=10  GraphicVisPropType=SimpleVisualProperties  GraphicDiffuseColor=[0.5 0.5 0.5]  GraphicOpacity=1.0  GraphicSpecularColor=[0.5 0.5 0.5 1.0]  GraphicAmbientColor=[0.15 0.15 0.15 1.0]  GraphicEmissiveColor=[0.0 0.0 0.0 1.0]  GraphicShininess=75  DoExposeReferenceFrame=on  SerializedFrames=<Frames/>
  World Frame : sm_lib/Frames and Transforms/World Frame
  basket_transform : sm_lib/Frames and Transforms/Rigid Transform  RotationMethod=None  FollAlignAxisA=+X  BaseAlignAxisA=+Y  FollAlignAxisB=+Y  BaseAlignAxisB=+Z  RotationStandardAxis=+Z  RotationAngle=0  RotationAngleUnits=deg  RotationArbitraryAxis=[0 0 1]  RotationSequenceAxes=FollowerAxes  RotationSequence=XYX  RotationSequenceAngles=[0 0 0]  RotationSequenceAnglesUnits=deg  RotationMatrix=[1 0 0;0 1 0;0 0 1]  Quaternion=[1 0 0 0]  TranslationMethod=Cartesian  TranslationCartesianOffset=[2.5, -1.9, 0]  TranslationCartesianOffsetUnits=m  TranslationStandardAxis=+Z  TranslationStandardOffset=0  TranslationStandardOffsetUnits=m  TranslationROffset=0  TranslationROffsetUnits=m  TranslationThetaOffset=0  TranslationThetaOffsetUnits=deg  TranslationZOffset=0  TranslationZOffsetUnits=m
  ball_x : PMIOPort  Side=Right
  ball_y : PMIOPort  Port=2  Side=Right
  ball_z : PMIOPort  Port=3  Side=Right
  shoulder_rot : PMIOPort  Port=4  Side=Right
  elbow_rot : PMIOPort  Port=5  Side=Right
  elbow_vel : PMIOPort  Port=6  Side=Right
  shoulder_vel : PMIOPort  Port=7  Side=Right
  elbow_rot_converted : Outport
  wires:
  PS-Simulink Converter1/1 -> Scope1/1, elbow_rot_converted/1
  PS-Simulink Converter/1 -> Scope/1
  elbow_torque/1 -> Simulink-PS Converter1/1
  shoulder_torque/1 -> Simulink-PS Converter/1
  connections:
  World Frame/RConn1 -- Shoulder Joint/LConn1 -- basket_transform/RConn1 -- Mechanism Configuration/RConn1 -- Rigid Transform3/LConn1 -- Transform Sensor/LConn1 -- Solver Configuration/RConn1
  Rigid Transform/LConn1 -- Shoulder Joint/RConn1
  Elbow Joint/RConn1 -- Rigid Transform2/LConn1
  PS-Simulink Converter1/LConn1 -- elbow_rot/RConn1 -- Elbow Joint/RConn2
  Rigid Transform4/RConn1 -- 6-DOF Joint/LConn1
  PS-Simulink Converter/LConn1 -- Shoulder Joint/RConn2 -- shoulder_rot/RConn1
  Elbow Joint/RConn3 -- elbow_vel/RConn1
  Rigid Transform3/RConn1 -- Rigid Transform4/LConn1
  6-DOF Joint/RConn1 -- Transform Sensor/RConn1 -- Spherical Solid/RConn1
  Rigid Transform1/LConn1 -- Upper Arm/RConn1 -- Rigid Transform/RConn1
  Spherical Solid/LConn1 -- Spatial Contact Force3/LConn1 -- Spatial Contact Force1/LConn1 -- Spatial Contact Force/LConn1
  Simulink-PS Converter1/RConn1 -- Elbow Joint/LConn2
  Lower Arm/LConn1 -- Spatial Contact Force/RConn1
  Elbow Joint/LConn1 -- Rigid Transform1/RConn1
  Rigid Transform2/RConn1 -- Lower Arm/RConn1
  Shoulder Joint/LConn2 -- Simulink-PS Converter/RConn1
  Shoulder Joint/RConn3 -- shoulder_vel/RConn1
  Spatial Contact Force1/RConn1 -- Upper Arm/LConn1
  Transform Sensor/RConn2 -- ball_x/RConn1
  Transform Sensor/RConn3 -- ball_y/RConn1
  Transform Sensor/RConn4 -- ball_z/RConn1
  Brick Solid1/RConn1 -- Rigid Transform5/LConn1
  Spatial Contact Force3/RConn1 -- Brick Solid1/LConn1
  Brick Solid/RConn1 -- Rigid Transform6/LConn1 -- Rigid Transform5/RConn1
  Rigid Transform6/RConn1 -- basket_transform/LConn1
